simulink model "rtwdemo_lct_cplxgain"  (Simulink 7.6)
settings: Solver=ode5  StartTime=0.0  StopTime=30  RelTol=1e-3  SampleTimeConstraint=STIndependent
libraries: rtwdemowidgets x2
Description:
  | Return Arguments
settings Model: Creator=The MathWorks Inc.  ExtModeAutoUpdateStatusClock=off
settings DataIOCC: SignalLoggingName=logsOut
settings OptimizationCC: InlineParams=on  InlineInvariantSignals=on  EfficientFloat2IntCast=on  EfficientMapNaN2IntZero=off
settings DebuggingCC: CheckExecutionContextPreStartOutputMsg=on  CheckExecutionContextRuntimeOutputMsg=on  SolverPrmCheckMsg=none  BusObjectLabelMismatch=error  StrictBusMsg=ErrorOnBusTreatedAsVector
settings HardwareCC: ProdIntDivRoundTo=Zero  ProdEndianess=LittleEndian  ProdHWDeviceType=Generic->32-bit Embedded Processor  TargetHWDeviceType=Generic->32-bit Embedded Processor
settings ModelReferenceCC: UpdateModelReferenceTargets=IfOutOfDate
settings RTWCC: TLCOptions=-p0 -aWarnNonSaturatedBlocks=0  GenerateReport=on  RTWVerbose=off  ProcessScript=grt_make_rtw_hook  LaunchReport=on
settings CodeAppCC: ForceParamTrailComments=on
settings GRTTargetCC: TargetFcnLib=ansi_tfl_tmw.mat

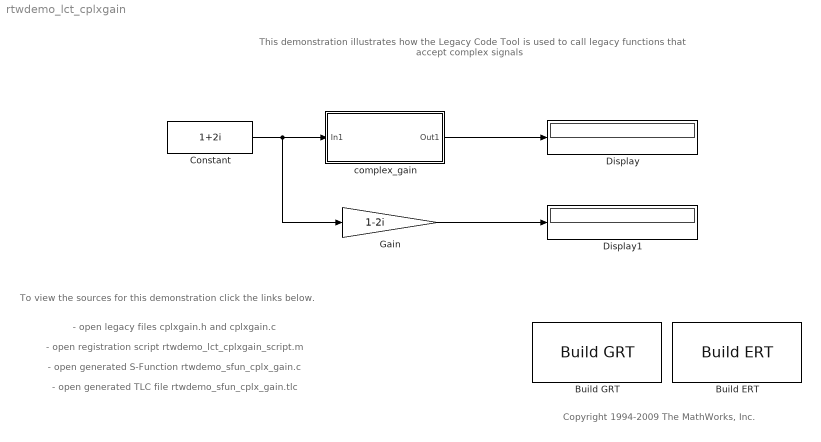
== system rtwdemo_lct_cplxgain ==
  note: This demonstration illustrates how the Legacy Code Tool is used to
      | call legacy functions that accept complex signals
  note: - open legacy files cplxgain.h and cplxgain.c
  note: To view the sources for this demonstration
      | click the links below.
  note: - open registration script rtwdemo_lct_cplxgain_script.m
  note: - open generated S-Function rtwdemo_sfun_cplx_gain.c
  note: Copyright 1994-2009 The MathWorks, Inc.
  note: - open generated TLC file rtwdemo_sfun_cplx_gain.tlc
  Build ERT : rtwdemowidgets/Build ERT  SystemSampleTime=-1  attrib_overrides={'SupportComplex'}
  Build GRT : rtwdemowidgets/Build GRT  SystemSampleTime=-1  attrib_overrides={}
  Constant : Constant  Value=1+2i
  Display : Display
  Display1 : Display
  Gain : Gain  Gain=1-2i
  complex_gain : Subsystem
  wires:
  complex_gain/1(Out1) -> Display/1
  Constant/1 -> complex_gain/1(In1), Gain/1
  Gain/1 -> Display1/1

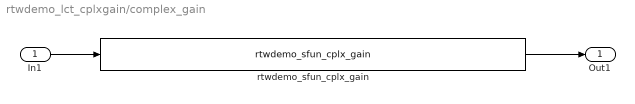
== system rtwdemo_lct_cplxgain/complex_gain ==
  In1 : Inport
  rtwdemo_sfun_cplx_gain : S-Function  FunctionName=rtwdemo_sfun_cplx_gain  Parameters=SParameter1  EnableBusSupport=off  mask(Legacy Function){SFunctionSpec=void cplx_gain(complex<double> u1[1], complex<double> p1[1], complex<double> y1[1]), SParameter1=1-2i, ShowSpec=on}
      mask prompts: SParameter1 "P1:"; ShowSpec "Display function specification"
      mask help:
      | This block allows you to call the legacy functions specified by the following Legacy Code Tool definition:
      | def.SFunctionName = 'rtwdemo_sfun_cplx_gain';
      | def.OutputFcnSpec = 'void cplx_gain(complex<double> u1[1], complex<double> p1[1], complex<double> y1[1])';
      | def.HeaderFiles = {'cplxgain.h'};
      | def.SourceFiles = {'cplxgain.c'};
      | def.IncPaths = {'sldemo_lct_src'};
      | def.SrcPaths = {'sldemo_lct_src'};
      mask Help: <p>This block was generated automatically by the Legacy Code Tool. For detailed help on this tool, call<a href="matlab:legacy_code('help')"> legacy_code('help')</a>.</p>
      mask CallbackString:
      | ||if strcmp(get_param(gcbh, 'ShowSpec'), 'on')
      |   set_param(gcbh, 'MaskDisplay', sprintf('fprintf(''%s'');', get_param(gcbh, 'SFunctionSpec')));
      | else
      |   set_param(gcbh, 'MaskDisplay', sprintf('fprintf(''%s'');', get_param(gcbh, 'FunctionName')));
      | end
      mask Display: fprintf('void cplx_gain(complex<double> u1[1], complex<double> p1[1], complex<double> y1[1])');
  Out1 : Outport
  wires:
  In1/1 -> rtwdemo_sfun_cplx_gain/1
  rtwdemo_sfun_cplx_gain/1 -> Out1/1
